simulink model "SimTest_Yitong"  (R2020b)
settings: Solver=FixedStepAuto  StartTime=0  StopTime=1  FixedStep=Ts  RelTol=1e-3
undefined symbols (not defined in the file or in its folder): Ts
libraries: SimplexPS x1, powerlib x1
settings Model: Creator=admin_user  LastModifiedBy=admin_user

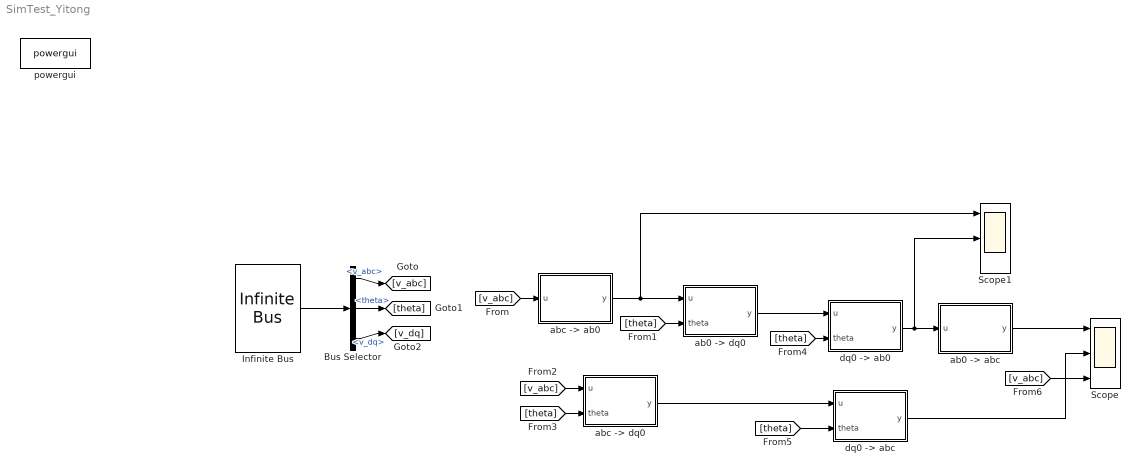
== system SimTest_Yitong ==
  Bus Selector : BusSelector  OutputSignals=v_abc,theta,v_dq
  Infinite Bus : SimplexPS/Infinite Bus  Ts=Ts  Sbase=Sbase  Vbase=Vbase  Wbase=Wbase  vd=1  vq=0  theta0=0  w=Wbase  R=1e-30
      settings: SourceProductName=Simplex Power Systems
  Scope : Scope  NumInputPorts=3
  Scope1 : Scope  NumInputPorts=3
  "ab0 -> abc" : MATLAB Function  TreatAsAtomicUnit=on
  "ab0 -> dq0" : MATLAB Function  TreatAsAtomicUnit=on
  "abc -> ab0" : MATLAB Function  TreatAsAtomicUnit=on
  "abc -> dq0" : MATLAB Function  TreatAsAtomicUnit=on
  "dq0 -> ab0" : MATLAB Function  TreatAsAtomicUnit=on
  "dq0 -> abc" : MATLAB Function  TreatAsAtomicUnit=on
  powergui : powerlib/powergui  Priority=1  SimulationMode=Discrete  SampleTime=Ts  frequency=60  Iterations=50  frequencyindice=0  Pbase=100e6  ErrMax=1e-4  UnitsV=kV  UnitsW=MW  buscounter=0  FunctionMessages=off  echomessages=off  EnableUseOfTLC=off  CurrentSourceSwitches=off  DisableSnubberDevices=off  DisableRonSwitches=off  DisableVfSwitches=off  DisplayEquations=off  AutomaticDiscreteSolvers=off  SolverType=Tustin/Backward Euler (TBE)  Interpol=off  ExternalGateDelay=off  methode=off  Ts=100  x0status=blocks  SPID=on  SwTol=0  HookPort=off  NonlinearTolerance=1e-4  nMaxIteration=100  ContinueOnMaxIteration=off  RestoreLinks=warning  ResistiveCurrentMeasurement=off  Frange=[0:2:500]  Ylog=off  Xlog=on  ShowGrid=off  save=off  variable=ZData  structure=0  ZoomFFT=off  StartTime=0.0  cycles=1  DisplayStyle=1  fundamental=60  FreqAxis=off  MaxFrequency=1000  frequencyindicesteady=1  RmsSteady=1  display=off
  wires:
  Infinite Bus/1 -> Bus Selector/1
  "abc -> ab0"/1(y) -> "ab0 -> dq0"/1(u), Scope1/1
  Bus Selector/1 -> [v_abc]  "<v_abc>"
  Bus Selector/2 -> [theta]  "<theta>"
  Bus Selector/3 -> [v_dq]  "<v_dq>"
  [v_abc] -> "abc -> ab0"/1(u)
  [theta] -> "ab0 -> dq0"/2(theta)
  [v_abc] -> "abc -> dq0"/1(u)
  [theta] -> "abc -> dq0"/2(theta)
  "dq0 -> abc"/1(y) -> Scope/2
  [theta] -> "dq0 -> ab0"/2(theta)
  [theta] -> "dq0 -> abc"/2(theta)
  "abc -> dq0"/1(y) -> "dq0 -> abc"/1(u)
  "ab0 -> dq0"/1(y) -> "dq0 -> ab0"/1(u)
  "dq0 -> ab0"/1(y) -> Scope1/2, "ab0 -> abc"/1(u)
  "ab0 -> abc"/1(y) -> Scope/1
  [v_abc] -> Scope/3

== matlab function SimTest_Yitong/abc -> ab0 ==
  data: u input; y output
function y = fcn(u)

y = SimplexPS.abc2alphabeta(u);

end

== matlab function SimTest_Yitong/abc -> dq0 ==
  data: u input; y output; theta input
function y = fcn(u,theta)

y = SimplexPS.abc2dq(u,theta,'PowerVariant',true);

end

== matlab function SimTest_Yitong/dq0 -> abc ==
  data: u input; y output; theta input
function y = fcn(u,theta)

y = SimplexPS.dq2abc(u,theta,'PowerVariant',true);

end

== matlab function SimTest_Yitong/dq0 -> ab0 ==
  data: u input; y output; theta input
function y = fcn(u,theta)

y = SimplexPS.dq2alphabeta(u,theta);

end

== matlab function SimTest_Yitong/ab0 -> abc ==
  data: u input; y output
function y = fcn(u)

y = SimplexPS.alphabeta2abc(u);

end

== matlab function SimTest_Yitong/ab0 -> dq0 ==
  data: u input; y output; theta input
function y = fcn(u,theta)

y = SimplexPS.alphabeta2dq(u,theta);

end
